simulink model "heli_ctrl"  (R2016a)
settings: Solver=FixedStepDiscrete  SolverMode=SingleTasking  StartTime=0.0  StopTime=inf  FixedStep=0.12345  RelTol=1e-3
undefined symbols (not defined in the file): gain_d, gain_i, gain_p
libraries: simulink x6
settings Model: Creator=Adam  LastModifiedBy=roussel
settings SolverCC: AutoInsertRateTranBlk=on
settings DataIOCC: SaveFormat=Array  SaveOutput=off  SignalLogging=off  DSMLogging=off  SaveTime=off
settings OptimizationCC: DefaultParameterBehavior=Inlined  DefaultUnderspecifiedDataType=single  InlineInvariantSignals=on  OptimizeModelRefInitCode=on  LifeSpan=Inf
settings DebuggingCC: SolverPrmCheckMsg=warning  UnconnectedInputMsg=none  UnconnectedOutputMsg=none  UnconnectedLineMsg=none  StateNameClashWarn=warning
settings HardwareCC: ProdBitPerPointer=32  ProdLargestAtomicInteger=Long  ProdIntDivRoundTo=Undefined  ProdWordSize=32  ProdHWDeviceType=ARM Compatible->ARM 7
settings ModelReferenceCC: PropagateSignalLabelsOutOfModel=off
settings RTWCC: SystemTargetFile=ert.tlc  GenCodeOnly=on  GenerateMakefile=off  TemplateMakefile=ert_default_tmf  RTWVerbose=off  CustomSourceCode=// User -- Source File  CustomHeaderCode=// User -- Header File  CustomInitializer=// User -- Initialize Function  CustomTerminator=// User -- Terminate Function  RTWCompilerOptimization=on
settings CodeAppCC: IgnoreCustomStorageClasses=off  SimulinkBlockComments=off  MATLABSourceComments=on
settings ERTTargetCC: SupportNonFinite=off  SupportComplex=off  ERTCustomFileTemplate=example_file_process.tlc  GlobalDataDefinition=InSourceFile  GlobalDataReference=InSourceFile  ERTFilePackagingFormat=Compact  ConvertIfToSwitch=off  PreserveExternInFcnDecls=off  SuppressUnreachableDefaultCases=off
settings ConfigComp: CovModelRefEnable=Off  CovSFcnEnable=off

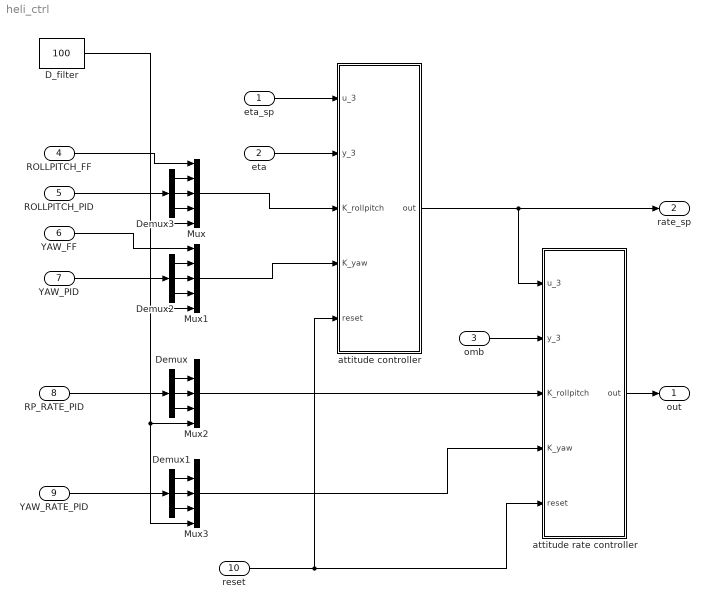
== system heli_ctrl ==
  eta_sp : Inport  OutDataTypeStr=single  PortDimensions=3  Interpolate=off
  eta : Inport  Port=2  OutDataTypeStr=single  PortDimensions=3  Interpolate=off
  omb : Inport  Port=3  OutDataTypeStr=single  PortDimensions=3  Interpolate=off
  ROLLPITCH_FF : Inport  Port=4  OutDataTypeStr=single  PortDimensions=1  Interpolate=off
  ROLLPITCH_PID : Inport  Port=5  OutDataTypeStr=single  PortDimensions=3  Interpolate=off
  YAW_FF : Inport  Port=6  OutDataTypeStr=single  PortDimensions=1  Interpolate=off
  YAW_PID : Inport  Port=7  OutDataTypeStr=single  PortDimensions=3  Interpolate=off
  RP_RATE_PID : Inport  Port=8  OutDataTypeStr=single  PortDimensions=3  Interpolate=off
  YAW_RATE_PID : Inport  Port=9  OutDataTypeStr=single  PortDimensions=3  Interpolate=off
  reset : Inport  Port=10  OutDataTypeStr=int8  PortDimensions=1  Interpolate=off
  D_filter : Constant  Value=100  OutDataTypeStr=single
  Demux{,1..3} (4 alike) : Demux  Outputs=3
  Mux{,1..3} (4 alike) : Mux  Inputs=5
  attitude controller : Subsystem
  attitude rate controller : Subsystem
  out : Outport
  rate_sp : Outport  Port=2
  wires:
  Mux/1 -> attitude controller/3(K_rollpitch)
  Mux1/1 -> attitude controller/4(K_yaw)
  attitude controller/1(out) -> attitude rate controller/1(u_3), rate_sp/1
  Mux2/1 -> attitude rate controller/3(K_rollpitch)
  Mux3/1 -> attitude rate controller/4(K_yaw)
  attitude rate controller/1(out) -> out/1
  D_filter/1 -> Mux3/5, Mux2/5, Mux1/5, Mux/5
  Demux/3 -> Mux2/4
  Demux/2 -> Mux2/3
  Demux/1 -> Mux2/2
  Demux1/1 -> Mux3/2
  Demux1/2 -> Mux3/3
  Demux1/3 -> Mux3/4
  Demux2/1 -> Mux1/2
  Demux2/2 -> Mux1/3
  Demux2/3 -> Mux1/4
  Demux3/1 -> Mux/2
  Demux3/2 -> Mux/3
  Demux3/3 -> Mux/4
  eta_sp/1 -> attitude controller/1(u_3)
  eta/1 -> attitude controller/2(y_3)
  omb/1 -> attitude rate controller/2(y_3)
  reset/1 -> attitude rate controller/5(reset), attitude controller/5(reset)
  YAW_RATE_PID/1 -> Demux1/1
  RP_RATE_PID/1 -> Demux/1
  YAW_PID/1 -> Demux2/1
  YAW_FF/1 -> Mux1/1
  ROLLPITCH_PID/1 -> Demux3/1
  ROLLPITCH_FF/1 -> Mux/1

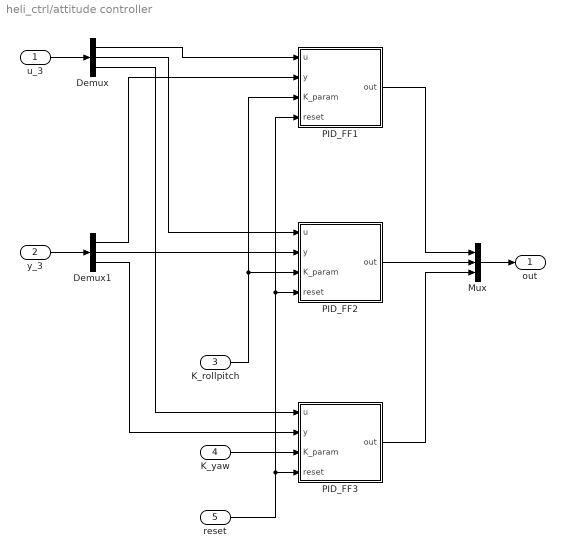
== system heli_ctrl/attitude controller ==
  u_3 : Inport
  y_3 : Inport  Port=2
  K_rollpitch : Inport  Port=3
  K_yaw : Inport  Port=4
  reset : Inport  Port=5
  Demux : Demux  Outputs=3
  Demux1 : Demux  Outputs=3
  Mux : Mux  Inputs=3
  PID_FF1 : Subsystem
  PID_FF2 : Subsystem
  PID_FF3 : Subsystem
  out : Outport
  wires:
  K_rollpitch/1 -> PID_FF1/3(K_param), PID_FF2/3(K_param)
  Mux/1 -> out/1
  PID_FF3/1(out) -> Mux/3
  PID_FF1/1(out) -> Mux/1
  reset/1 -> PID_FF1/4(reset), PID_FF2/4(reset), PID_FF3/4(reset)
  K_yaw/1 -> PID_FF3/3(K_param)
  Demux1/1 -> PID_FF1/2(y)
  PID_FF2/1(out) -> Mux/2
  y_3/1 -> Demux1/1
  Demux/1 -> PID_FF1/1(u)
  u_3/1 -> Demux/1
  Demux1/2 -> PID_FF2/2(y)
  Demux1/3 -> PID_FF3/2(y)
  Demux/2 -> PID_FF2/1(u)
  Demux/3 -> PID_FF3/1(u)

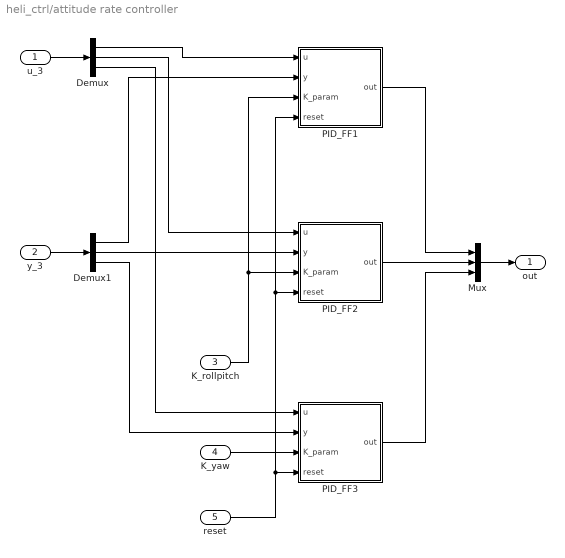
== system heli_ctrl/attitude rate controller ==
  u_3 : Inport
  y_3 : Inport  Port=2
  K_rollpitch : Inport  Port=3
  K_yaw : Inport  Port=4
  reset : Inport  Port=5
  Demux : Demux  Outputs=3
  Demux1 : Demux  Outputs=3
  Mux : Mux  Inputs=3
  PID_FF1 : Subsystem
  PID_FF2 : Subsystem
  PID_FF3 : Subsystem
  out : Outport
  wires:
  K_rollpitch/1 -> PID_FF1/3(K_param), PID_FF2/3(K_param)
  Mux/1 -> out/1
  PID_FF3/1(out) -> Mux/3
  PID_FF1/1(out) -> Mux/1
  reset/1 -> PID_FF1/4(reset), PID_FF2/4(reset), PID_FF3/4(reset)
  K_yaw/1 -> PID_FF3/3(K_param)
  Demux1/1 -> PID_FF1/2(y)
  PID_FF2/1(out) -> Mux/2
  y_3/1 -> Demux1/1
  Demux/1 -> PID_FF1/1(u)
  u_3/1 -> Demux/1
  Demux1/2 -> PID_FF2/2(y)
  Demux1/3 -> PID_FF3/2(y)
  Demux/2 -> PID_FF2/1(u)
  Demux/3 -> PID_FF3/1(u)

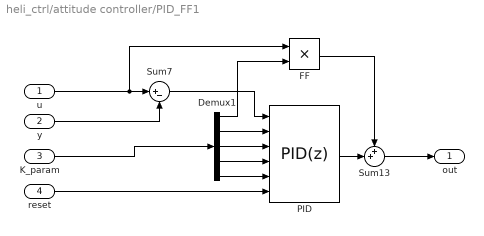
== system heli_ctrl/attitude controller/PID_FF1 ==
  u : Inport
  y : Inport  Port=2
  K_param : Inport  Port=3
  reset : Inport  Port=4
  Demux1 : Demux  Outputs=5
  FF : Product
  PID : simulink/Continuous/PID Controller  Controller=PID  TimeDomain=Discrete-time  SampleTime=-1  IntegratorMethod=Forward Euler  FilterMethod=Forward Euler  Form=Parallel  UseFilter=on  ControllerParametersSource=external  P=gain_p  I=gain_i  D=gain_d  N=100  InitialConditionSource=internal  InitialConditionForIntegrator=0  InitialConditionForFilter=0  ExternalReset=level  LimitOutput=off  UpperSaturationLimit=1  LowerSaturationLimit=-1  LinearizeAsGain=on  AntiWindupMode=back-calculation  Kb=1  TrackingMode=off  Kt=1  PParamMin=[]  PParamMax=[]  IParamMin=[]  IParamMax=[]  DParamMin=[]  DParamMax=[]  NParamMin=[]  NParamMax=[]  KbParamMin=[]  KbParamMax=[]  KtParamMin=[]  KtParamMax=[]  POutMin=[]  POutMax=[]  IOutMin=[]  IOutMax=[]  DOutMin=[]  DOutMax=[]  NOutMin=[]  NOutMax=[]  KbOutMin=[]  KbOutMax=[]  KtOutMin=[]  KtOutMax=[]  IntegratorOutMin=[]  IntegratorOutMax=[]  FilterOutMin=[]  FilterOutMax=[]  SumOutMin=[]  SumOutMax=[]  SumI1OutMin=[]  SumI1OutMax=[]  SumI2OutMin=[]  SumI2OutMax=[]  SumI3OutMin=[]  SumI3OutMax=[]  SumDOutMin=[]  SumDOutMax=[]  SaturationOutMin=[]  SaturationOutMax=[]  IntegratorContinuousStateAttributes=''  IntegratorStateMustResolveToSignalObject=off  IntegratorRTWStateStorageClass=Auto  FilterContinuousStateAttributes=''  FilterStateMustResolveToSignalObject=off  FilterRTWStateStorageClass=Auto  DifferentiatorICPrevScaledInput=0  DifferentiatorOutMin=[]  DifferentiatorOutMax=[]
  Sum13 : Sum  Inputs=++|
  Sum7 : Sum  Inputs=|+-
  out : Outport
  wires:
  Demux1/3 -> PID/3
  K_param/1 -> Demux1/1
  Demux1/2 -> PID/2
  FF/1 -> Sum13/1
  Sum13/1 -> out/1
  Sum7/1 -> PID/1
  PID/1 -> Sum13/2
  Demux1/5 -> PID/5
  reset/1 -> PID/6
  Demux1/4 -> PID/4
  u/1 -> FF/1, Sum7/1
  y/1 -> Sum7/2
  Demux1/1 -> FF/2

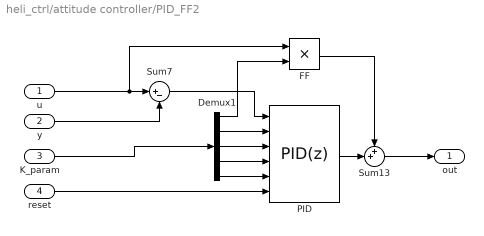
== system heli_ctrl/attitude controller/PID_FF2 ==
  u : Inport
  y : Inport  Port=2
  K_param : Inport  Port=3
  reset : Inport  Port=4
  Demux1 : Demux  Outputs=5
  FF : Product
  PID : simulink/Continuous/PID Controller  Controller=PID  TimeDomain=Discrete-time  SampleTime=-1  IntegratorMethod=Forward Euler  FilterMethod=Forward Euler  Form=Parallel  UseFilter=on  ControllerParametersSource=external  P=gain_p  I=gain_i  D=gain_d  N=100  InitialConditionSource=internal  InitialConditionForIntegrator=0  InitialConditionForFilter=0  ExternalReset=level  LimitOutput=off  UpperSaturationLimit=1  LowerSaturationLimit=-1  LinearizeAsGain=on  AntiWindupMode=back-calculation  Kb=1  TrackingMode=off  Kt=1  PParamMin=[]  PParamMax=[]  IParamMin=[]  IParamMax=[]  DParamMin=[]  DParamMax=[]  NParamMin=[]  NParamMax=[]  KbParamMin=[]  KbParamMax=[]  KtParamMin=[]  KtParamMax=[]  POutMin=[]  POutMax=[]  IOutMin=[]  IOutMax=[]  DOutMin=[]  DOutMax=[]  NOutMin=[]  NOutMax=[]  KbOutMin=[]  KbOutMax=[]  KtOutMin=[]  KtOutMax=[]  IntegratorOutMin=[]  IntegratorOutMax=[]  FilterOutMin=[]  FilterOutMax=[]  SumOutMin=[]  SumOutMax=[]  SumI1OutMin=[]  SumI1OutMax=[]  SumI2OutMin=[]  SumI2OutMax=[]  SumI3OutMin=[]  SumI3OutMax=[]  SumDOutMin=[]  SumDOutMax=[]  SaturationOutMin=[]  SaturationOutMax=[]  IntegratorContinuousStateAttributes=''  IntegratorStateMustResolveToSignalObject=off  IntegratorRTWStateStorageClass=Auto  FilterContinuousStateAttributes=''  FilterStateMustResolveToSignalObject=off  FilterRTWStateStorageClass=Auto  DifferentiatorICPrevScaledInput=0  DifferentiatorOutMin=[]  DifferentiatorOutMax=[]
  Sum13 : Sum  Inputs=++|
  Sum7 : Sum  Inputs=|+-
  out : Outport
  wires:
  Demux1/3 -> PID/3
  K_param/1 -> Demux1/1
  Demux1/2 -> PID/2
  FF/1 -> Sum13/1
  Sum13/1 -> out/1
  Sum7/1 -> PID/1
  PID/1 -> Sum13/2
  Demux1/5 -> PID/5
  reset/1 -> PID/6
  Demux1/4 -> PID/4
  u/1 -> FF/1, Sum7/1
  y/1 -> Sum7/2
  Demux1/1 -> FF/2

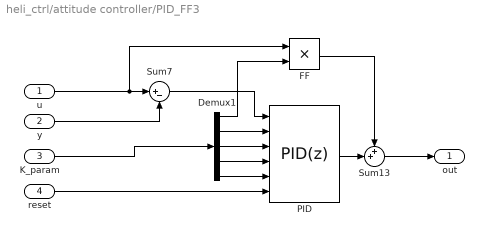
== system heli_ctrl/attitude controller/PID_FF3 ==
  u : Inport
  y : Inport  Port=2
  K_param : Inport  Port=3
  reset : Inport  Port=4
  Demux1 : Demux  Outputs=5
  FF : Product
  PID : simulink/Continuous/PID Controller  Controller=PID  TimeDomain=Discrete-time  SampleTime=-1  IntegratorMethod=Forward Euler  FilterMethod=Forward Euler  Form=Parallel  UseFilter=on  ControllerParametersSource=external  P=gain_p  I=gain_i  D=gain_d  N=100  InitialConditionSource=internal  InitialConditionForIntegrator=0  InitialConditionForFilter=0  ExternalReset=level  LimitOutput=off  UpperSaturationLimit=1  LowerSaturationLimit=-1  LinearizeAsGain=on  AntiWindupMode=back-calculation  Kb=1  TrackingMode=off  Kt=1  PParamMin=[]  PParamMax=[]  IParamMin=[]  IParamMax=[]  DParamMin=[]  DParamMax=[]  NParamMin=[]  NParamMax=[]  KbParamMin=[]  KbParamMax=[]  KtParamMin=[]  KtParamMax=[]  POutMin=[]  POutMax=[]  IOutMin=[]  IOutMax=[]  DOutMin=[]  DOutMax=[]  NOutMin=[]  NOutMax=[]  KbOutMin=[]  KbOutMax=[]  KtOutMin=[]  KtOutMax=[]  IntegratorOutMin=[]  IntegratorOutMax=[]  FilterOutMin=[]  FilterOutMax=[]  SumOutMin=[]  SumOutMax=[]  SumI1OutMin=[]  SumI1OutMax=[]  SumI2OutMin=[]  SumI2OutMax=[]  SumI3OutMin=[]  SumI3OutMax=[]  SumDOutMin=[]  SumDOutMax=[]  SaturationOutMin=[]  SaturationOutMax=[]  IntegratorContinuousStateAttributes=''  IntegratorStateMustResolveToSignalObject=off  IntegratorRTWStateStorageClass=Auto  FilterContinuousStateAttributes=''  FilterStateMustResolveToSignalObject=off  FilterRTWStateStorageClass=Auto  DifferentiatorICPrevScaledInput=0  DifferentiatorOutMin=[]  DifferentiatorOutMax=[]
  Sum13 : Sum  Inputs=++|
  Sum7 : Sum  Inputs=|+-
  out : Outport
  wires:
  Demux1/3 -> PID/3
  K_param/1 -> Demux1/1
  Demux1/2 -> PID/2
  FF/1 -> Sum13/1
  Sum13/1 -> out/1
  Sum7/1 -> PID/1
  PID/1 -> Sum13/2
  Demux1/5 -> PID/5
  reset/1 -> PID/6
  Demux1/4 -> PID/4
  u/1 -> FF/1, Sum7/1
  y/1 -> Sum7/2
  Demux1/1 -> FF/2

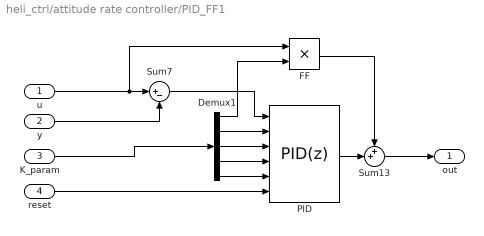
== system heli_ctrl/attitude rate controller/PID_FF1 ==
  u : Inport
  y : Inport  Port=2
  K_param : Inport  Port=3
  reset : Inport  Port=4
  Demux1 : Demux  Outputs=5
  FF : Product
  PID : simulink/Continuous/PID Controller  Controller=PID  TimeDomain=Discrete-time  SampleTime=-1  IntegratorMethod=Forward Euler  FilterMethod=Forward Euler  Form=Parallel  UseFilter=on  ControllerParametersSource=external  P=gain_p  I=gain_i  D=gain_d  N=100  InitialConditionSource=internal  InitialConditionForIntegrator=0  InitialConditionForFilter=0  ExternalReset=level  LimitOutput=off  UpperSaturationLimit=1  LowerSaturationLimit=-1  LinearizeAsGain=on  AntiWindupMode=back-calculation  Kb=1  TrackingMode=off  Kt=1  PParamMin=[]  PParamMax=[]  IParamMin=[]  IParamMax=[]  DParamMin=[]  DParamMax=[]  NParamMin=[]  NParamMax=[]  KbParamMin=[]  KbParamMax=[]  KtParamMin=[]  KtParamMax=[]  POutMin=[]  POutMax=[]  IOutMin=[]  IOutMax=[]  DOutMin=[]  DOutMax=[]  NOutMin=[]  NOutMax=[]  KbOutMin=[]  KbOutMax=[]  KtOutMin=[]  KtOutMax=[]  IntegratorOutMin=[]  IntegratorOutMax=[]  FilterOutMin=[]  FilterOutMax=[]  SumOutMin=[]  SumOutMax=[]  SumI1OutMin=[]  SumI1OutMax=[]  SumI2OutMin=[]  SumI2OutMax=[]  SumI3OutMin=[]  SumI3OutMax=[]  SumDOutMin=[]  SumDOutMax=[]  SaturationOutMin=[]  SaturationOutMax=[]  IntegratorContinuousStateAttributes=''  IntegratorStateMustResolveToSignalObject=off  IntegratorRTWStateStorageClass=Auto  FilterContinuousStateAttributes=''  FilterStateMustResolveToSignalObject=off  FilterRTWStateStorageClass=Auto  DifferentiatorICPrevScaledInput=0  DifferentiatorOutMin=[]  DifferentiatorOutMax=[]
  Sum13 : Sum  Inputs=++|
  Sum7 : Sum  Inputs=|+-
  out : Outport
  wires:
  Demux1/3 -> PID/3
  K_param/1 -> Demux1/1
  Demux1/2 -> PID/2
  FF/1 -> Sum13/1
  Sum13/1 -> out/1
  Sum7/1 -> PID/1
  PID/1 -> Sum13/2
  Demux1/5 -> PID/5
  reset/1 -> PID/6
  Demux1/4 -> PID/4
  u/1 -> FF/1, Sum7/1
  y/1 -> Sum7/2
  Demux1/1 -> FF/2

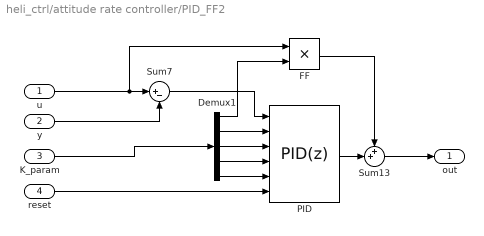
== system heli_ctrl/attitude rate controller/PID_FF2 ==
  u : Inport
  y : Inport  Port=2
  K_param : Inport  Port=3
  reset : Inport  Port=4
  Demux1 : Demux  Outputs=5
  FF : Product
  PID : simulink/Continuous/PID Controller  Controller=PID  TimeDomain=Discrete-time  SampleTime=-1  IntegratorMethod=Forward Euler  FilterMethod=Forward Euler  Form=Parallel  UseFilter=on  ControllerParametersSource=external  P=gain_p  I=gain_i  D=gain_d  N=100  InitialConditionSource=internal  InitialConditionForIntegrator=0  InitialConditionForFilter=0  ExternalReset=level  LimitOutput=off  UpperSaturationLimit=1  LowerSaturationLimit=-1  LinearizeAsGain=on  AntiWindupMode=back-calculation  Kb=1  TrackingMode=off  Kt=1  PParamMin=[]  PParamMax=[]  IParamMin=[]  IParamMax=[]  DParamMin=[]  DParamMax=[]  NParamMin=[]  NParamMax=[]  KbParamMin=[]  KbParamMax=[]  KtParamMin=[]  KtParamMax=[]  POutMin=[]  POutMax=[]  IOutMin=[]  IOutMax=[]  DOutMin=[]  DOutMax=[]  NOutMin=[]  NOutMax=[]  KbOutMin=[]  KbOutMax=[]  KtOutMin=[]  KtOutMax=[]  IntegratorOutMin=[]  IntegratorOutMax=[]  FilterOutMin=[]  FilterOutMax=[]  SumOutMin=[]  SumOutMax=[]  SumI1OutMin=[]  SumI1OutMax=[]  SumI2OutMin=[]  SumI2OutMax=[]  SumI3OutMin=[]  SumI3OutMax=[]  SumDOutMin=[]  SumDOutMax=[]  SaturationOutMin=[]  SaturationOutMax=[]  IntegratorContinuousStateAttributes=''  IntegratorStateMustResolveToSignalObject=off  IntegratorRTWStateStorageClass=Auto  FilterContinuousStateAttributes=''  FilterStateMustResolveToSignalObject=off  FilterRTWStateStorageClass=Auto  DifferentiatorICPrevScaledInput=0  DifferentiatorOutMin=[]  DifferentiatorOutMax=[]
  Sum13 : Sum  Inputs=++|
  Sum7 : Sum  Inputs=|+-
  out : Outport
  wires:
  Demux1/3 -> PID/3
  K_param/1 -> Demux1/1
  Demux1/2 -> PID/2
  FF/1 -> Sum13/1
  Sum13/1 -> out/1
  Sum7/1 -> PID/1
  PID/1 -> Sum13/2
  Demux1/5 -> PID/5
  reset/1 -> PID/6
  Demux1/4 -> PID/4
  u/1 -> FF/1, Sum7/1
  y/1 -> Sum7/2
  Demux1/1 -> FF/2

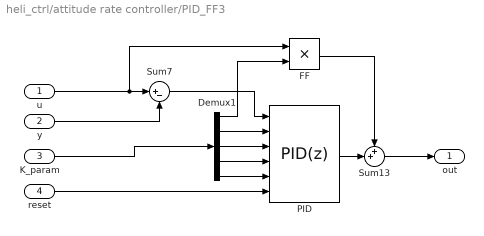
== system heli_ctrl/attitude rate controller/PID_FF3 ==
  u : Inport
  y : Inport  Port=2
  K_param : Inport  Port=3
  reset : Inport  Port=4
  Demux1 : Demux  Outputs=5
  FF : Product
  PID : simulink/Continuous/PID Controller  Controller=PID  TimeDomain=Discrete-time  SampleTime=-1  IntegratorMethod=Forward Euler  FilterMethod=Forward Euler  Form=Parallel  UseFilter=on  ControllerParametersSource=external  P=gain_p  I=gain_i  D=gain_d  N=100  InitialConditionSource=internal  InitialConditionForIntegrator=0  InitialConditionForFilter=0  ExternalReset=level  LimitOutput=off  UpperSaturationLimit=1  LowerSaturationLimit=-1  LinearizeAsGain=on  AntiWindupMode=back-calculation  Kb=1  TrackingMode=off  Kt=1  PParamMin=[]  PParamMax=[]  IParamMin=[]  IParamMax=[]  DParamMin=[]  DParamMax=[]  NParamMin=[]  NParamMax=[]  KbParamMin=[]  KbParamMax=[]  KtParamMin=[]  KtParamMax=[]  POutMin=[]  POutMax=[]  IOutMin=[]  IOutMax=[]  DOutMin=[]  DOutMax=[]  NOutMin=[]  NOutMax=[]  KbOutMin=[]  KbOutMax=[]  KtOutMin=[]  KtOutMax=[]  IntegratorOutMin=[]  IntegratorOutMax=[]  FilterOutMin=[]  FilterOutMax=[]  SumOutMin=[]  SumOutMax=[]  SumI1OutMin=[]  SumI1OutMax=[]  SumI2OutMin=[]  SumI2OutMax=[]  SumI3OutMin=[]  SumI3OutMax=[]  SumDOutMin=[]  SumDOutMax=[]  SaturationOutMin=[]  SaturationOutMax=[]  IntegratorContinuousStateAttributes=''  IntegratorStateMustResolveToSignalObject=off  IntegratorRTWStateStorageClass=Auto  FilterContinuousStateAttributes=''  FilterStateMustResolveToSignalObject=off  FilterRTWStateStorageClass=Auto  DifferentiatorICPrevScaledInput=0  DifferentiatorOutMin=[]  DifferentiatorOutMax=[]
  Sum13 : Sum  Inputs=++|
  Sum7 : Sum  Inputs=|+-
  out : Outport
  wires:
  Demux1/3 -> PID/3
  K_param/1 -> Demux1/1
  Demux1/2 -> PID/2
  FF/1 -> Sum13/1
  Sum13/1 -> out/1
  Sum7/1 -> PID/1
  PID/1 -> Sum13/2
  Demux1/5 -> PID/5
  reset/1 -> PID/6
  Demux1/4 -> PID/4
  u/1 -> FF/1, Sum7/1
  y/1 -> Sum7/2
  Demux1/1 -> FF/2
